simulink library "libAeroCoeffCalcs"  (R2020b)
settings: Solver=VariableStepAuto  StartTime=0.0  StopTime=10.0  RelTol=1e-3
undefined symbols (not defined in the file): data
libraries: aerolibconvert2 x2
settings Model: Creator=caatay  LastModifiedBy=caatay

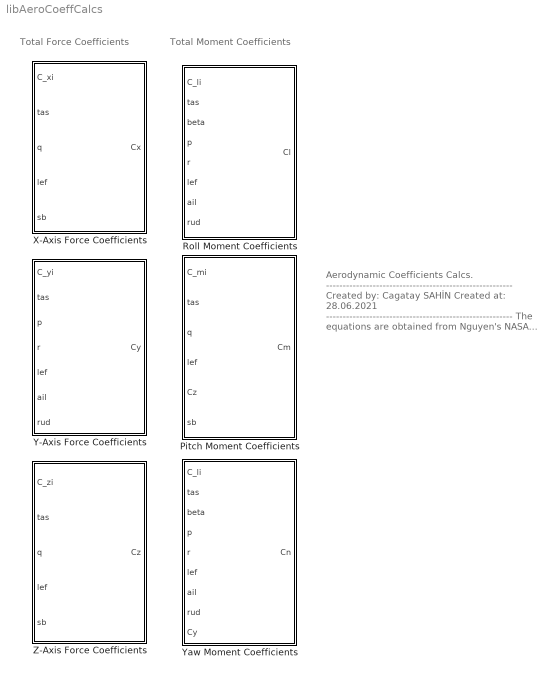
== system libAeroCoeffCalcs ==
  note: Aerodynamic Coefficients Calcs.
      | --------------------------------------------------------
      | Created by: Cagatay SAHİN
      | Created at: 28.06.2021
      | --------------------------------------------------------
      | The equations are obtained from
      | Nguyen's NASA works.
      | The reference article can be found in
      | "references folder".
      | --------------------------------------------------------
      | for question:
      | cagataysahin44@gmail.com
  note: Total Moment Coefficients
  note: Total Force Coefficients
  Pitch Moment Coefficients : Subsystem  mask(Aerodynamic Model - Total Coefficient Calculations - Total Pitch Moment Body Aerodynamic Coefficient){cbar=data.acSpec.wing.cbar, xcg=data.acSpec.fusalage.x_cg, xcg_ref=data.acSpec.fusalage.x_cg_ref}
      mask prompts: cbar "Mean Aerodynamic Chord"; xcg "X-axis center of gravity"; xcg_ref "Nominal X-axis center of gravity"
      mask help: Aircraft's total pitch moment aerodynamic coefficient calculations with using state variables and control inputs.
      mask Help:
      | This block is used for obtain total pitch moment coefficient with using state and control inputs.
      | -------------------------------------------------------------------------------------------------------------------------------------------------
      | Inputs of the function:
      | 	Coefficients C_{m}s: Pitch Moment whole aerodynamic coefficients at specific conditions.
      | 	tas: True air speed in [ft/s].
      | 	q: Body axis angular rate (pitch) in [rad/s].
      | 	lef: Leading edge flap deflection in [deg].
      | 	C_{z}: Z-Axis total aeodynamic coefficient.
      | Output of the function:
      | 	C_{m}: Pitch Moment total aerodynamic coefficient.
      | -------------------------------------------------------------------------------------------------------------------------------------------------
      | All equations can be found in Steven's text book. Reference can be found in "literature" subfolder.
      | for question: "cagataysahin44@gmail.com"
      mask Display:
      | port_label('input',1,'C_{m_{i}}','texmode','on');
      | port_label('input',2,'V_{tas}','texmode','on');
      | port_label('input',3,'q','texmode','on');
      | port_label('input',4,'\delta_{lef}','texmode','on');
      | port_label('input',5,'C_{z}','texmode','on');
      | port_label('input',6,'\delta_{sb}','texmode','on');
      | 
      | port_label('output',1,'C_{m}','texmode','on');
  Roll Moment Coefficients : Subsystem  mask(Aerodynamic Model - Total Coefficient Calculations - Total Roll Moment Body Aerodynamic Coefficient){b=data.acSpec.wing.b}
      mask prompts: b "Wing Span"
      mask help: Aircraft's total roll moment aerodynamic coefficient calculations with using state variables and control input
      mask Help:
      | This block is used for obtain total roll moment aerodynamic force coefficient. The equations are taken from Steven's textbook.,
      | -------------------------------------------------------------------------------------------------------------------------------------------------
      | Inputs of the function:
      | 	Coefficients C_{l}s: Roll moment whole aerodynamic coefficients at specific conditions.
      | 	tas: True air speed in [ft/s].
      |  	beta: Sideslip angle in [rad].
      | 	p: Body axis angular rate (roll) in [rad/s].
      | 	r: Body axis angular rate (yaw) in [rad/s].
      | 	lef: Leading edge flap deflection in [deg].
      | 	ail: Aileron deflection in [deg].
      | 	rud: Rudder deflection in [deg].
      | Output of the function:
      | 	C_{l}: Roll moment aerodynamic coefficient.
      | -------------------------------------------------------------------------------------------------------------------------------------------------
      | All equations can be found in Steven's text book. Reference can be found in "literature" subfolder.
      | for question: "cagataysahin44@gmail.com"
      mask Display:
      | port_label('input',1,'C_{l_{i}}','texmode','on');
      | port_label('input',2,'V_{tas}','texmode','on');
      | port_label('input',3,'\beta','texmode','on');
      | port_label('input',4,'p','texmode','on');
      | port_label('input',5,'r','texmode','on');
      | port_label('input',6,'\delta_{lef}','texmode','on');
      | port_label('input',7,'\delta_{ail}','texmode','on');
      | port_label('input',8,'\delta_{rud}','texmode','on');
      | 
      | port_label('output',1,'C_{l}','texmode','on');
  X-Axis Force Coefficients : Subsystem  mask(Aerodynamic Model - Total Coefficient Calculations - Total X-Axis Body Aerodynamic Coefficient){cbar=data.acSpec.wing.cbar}
      mask prompts: cbar "Mean Aerodynamic Chord"
      mask help: Aircraft's total X-Axis aerodynamic coefficient calculations with using state variables and control inputs.
      mask Help:
      | This block is used for obtain total x-axis aerodynamic force coefficient with using state and control inputs.
      | -------------------------------------------------------------------------------------------------------------------------------------------------
      | Inputs of the function:
      | 	Coefficients C_{x}s: X-Axis whole aerodynamic coefficients at specific conditions.
      | 	tas: True air speed in [ft/s].
      | 	q: Body axis angular rate (pitch) in [rad/s].
      | 	lef: Leading edge flap deflection in [deg].
      | Output of the function:
      | 	C_{x}: X-Axis total aerodynamic coefficient.
      | -------------------------------------------------------------------------------------------------------------------------------------------------
      | All equations can be found in Steven's text book. Reference can be found in "literature" subfolder.
      | for question: "cagataysahin44@gmail.com"
      mask Display:
      | port_label('input',1,'C_{x_{i}}','texmode','on');
      | port_label('input',2,'V_{tas}','texmode','on');
      | port_label('input',3,'q','texmode','on');
      | port_label('input',4,'\delta_{lef}','texmode','on');
      | port_label('input',5,'\delta_{sb}','texmode','on');
      | 
      | port_label('output',1,'C_{x}','texmode','on');
  Y-Axis Force Coefficients : Subsystem  mask(Aerodynamic Model - Total Coefficient Calculations - Total Y-Axis Body Aerodynamic Coefficient){b=data.acSpec.wing.b}
      mask prompts: b "Wing Span"
      mask help: Aircraft's total Y-Axis aerodynamic coefficient calculations with using state variables and control inputs.
      mask Help:
      | This block is used for obtain total x-axis aerodynamic force coefficient with using state and control inputs.
      | -------------------------------------------------------------------------------------------------------------------------------------------------
      | Inputs of the function:
      | 	Coefficients C_{y}s: Y-Axis whole aerodynamic coefficients at specific conditions.
      | 	tas: True air speed in [ft/s].
      | 	p: Body axis angular rate (y-axis) in [rad/s].
      | 	r: Body axis angular rate (y-axis) in [rad/s].
      | 	lef: Leading edge flap deflection in [deg].
      | 	ail: Aileron deflection in [deg].
      | 	rud: Rudder deflection in [deg].
      | Output of the function:
      | 	C_{y}: Y-axis total aerodynamic coefficient.
      | -------------------------------------------------------------------------------------------------------------------------------------------------
      | All equations can be found in Steven's text book. Reference can be found in "literature" subfolder.
      | for question: "cagataysahin44@gmail.com"
      mask Display:
      | port_label('input',1,'C_{y_{i}}','texmode','on');
      | port_label('input',2,'V_{tas}','texmode','on');
      | port_label('input',3,'p','texmode','on');
      | port_label('input',4,'r','texmode','on');
      | port_label('input',5,'\delta_{lef}','texmode','on');
      | port_label('input',6,'\delta_{ail}','texmode','on');
      | port_label('input',7,'\delta_{rud}','texmode','on');
      | 
      | port_label('output',1,'C_{y}','texmode','on');
  Yaw Moment Coefficients : Subsystem  mask(Aerodynamic Model - Total Coefficient Calculations - Total Yaw Moment Body Aerodynamic Coefficient){b=data.acSpec.wing.b, xcg=data.acSpec.fusalage.x_cg, xcg_ref=data.acSpec.fusalage.x_cg_ref, cbar=data.acSpec.wing.cbar}
      mask prompts: b "Wing Span"; xcg "Center of Gravity"; xcg_ref "Nominal Center of Gravity"; cbar "Mean Aerodynamic Chord"
      mask help: Aircraft's total yaw moment aerodynamic coefficient calculations with using state variables and control inputs.
      mask Help:
      | This block is used for obtain total yaw moment aerodynamic force coefficient. The equations are taken from Steven's textbook.,
      | -------------------------------------------------------------------------------------------------------------------------------------------------
      | Inputs of the function:
      | 	Coefficients C_{n}s: Yaw moment whole aerodynamic coefficients at specific conditions.
      | 	tas: True air speed in [ft/s].
      |  	beta: Sideslip angle in [rad].
      | 	p: Body axis angular rate (roll) in [rad/s].
      | 	r: Body axis angular rate (yaw) in [rad/s].
      | 	lef: Leading edge flap deflection in [deg].
      | 	ail: Aileron deflection in [deg].
      | 	rud: Rudder deflection in [deg].
      | 	C_{y}: Total Y-Axis aerodynamic coefficient.
      | Output of the function:
      | 	C_{n}: Yaw moment aerodynamic coefficient.
      | -------------------------------------------------------------------------------------------------------------------------------------------------
      | All equations can be found in Steven's text book. Reference can be found in "literature" subfolder.
      | for question: "cagataysahin44@gmail.com"
      mask Display:
      | port_label('input',1,'C_{n_{i}}','texmode','on');
      | port_label('input',2,'V_{tas}','texmode','on');
      | port_label('input',3,'\beta','texmode','on');
      | port_label('input',4,'p','texmode','on');
      | port_label('input',5,'r','texmode','on');
      | port_label('input',6,'\delta_{lef}','texmode','on');
      | port_label('input',7,'\delta_{ail}','texmode','on');
      | port_label('input',8,'\delta_{rud}','texmode','on');
      | port_label('input',9,'C_{y}','texmode','on');
      | 
      | port_label('output',1,'C_{n}','texmode','on');
  Z-Axis Force Coefficients : Subsystem  mask(Aerodynamic Model - Total Coefficient Calculations - Total Z-Axis Body Aerodynamic Coefficient){cbar=data.acSpec.wing.cbar}
      mask prompts: cbar "Mean Aerodynamic Chord"
      mask help: Aircraft's total Z-Axis aerodynamic coefficient calculations with using state variables and control inputs.
      mask Help:
      | This block is used for obtain total z-axis aerodynamic force coefficient with using state and control inputs.
      | -------------------------------------------------------------------------------------------------------------------------------------------------
      | Inputs of the function:
      | 	Coefficients C_{z}s: Z-Axis whole aerodynamic coefficients at specific conditions.
      | 	tas: True air speed in [ft/s].
      | 	q: Body axis angular rate (pitch) in [rad/s].
      | 	lef: Leading edge flap deflection in [deg].
      | Output of the function:
      | 	C_{z}: X-Axis total aerodynamic coefficient.
      | -------------------------------------------------------------------------------------------------------------------------------------------------
      | All equations can be found in Steven's text book. Reference can be found in "literature" subfolder.
      | for question: "cagataysahin44@gmail.com"
      mask Display:
      | port_label('input',1,'C_{z_{i}}','texmode','on');
      | port_label('input',2,'V_{tas}','texmode','on');
      | port_label('input',3,'q','texmode','on');
      | port_label('input',4,'\delta_{lef}','texmode','on');
      | port_label('input',5,'\delta_{sb}','texmode','on');
      | 
      | port_label('output',1,'C_{z}','texmode','on');

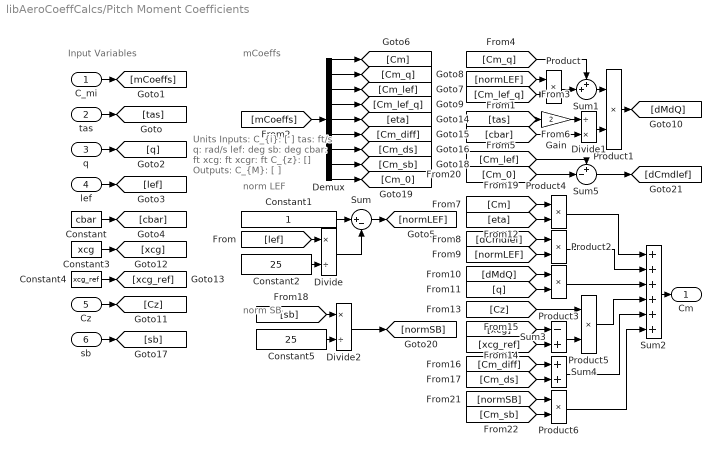
== system libAeroCoeffCalcs/Pitch Moment Coefficients ==
  note: Units
      | Inputs:
      | C_{i}: [ ]
      | tas: ft/s
      | q: rad/s
      | lef: deg
      | sb: deg
      | cbar: ft
      | xcg: ft
      | xcgr: ft
      | C_{z}: []
      | Outputs:
      | C_{M}: [ ]
  note: mCoeffs
  note: Input Variables
  note: norm LEF
  note: norm SB
  C_mi : Inport
  tas : Inport  Port=2
  q : Inport  Port=3
  lef : Inport  Port=4
  Cz : Inport  Port=5
  sb : Inport  Port=6
  Constant : Constant  Value=cbar
  Constant1 : Constant
  Constant2 : Constant  Value=25
  Constant3 : Constant  Value=xcg
  Constant4 : Constant  Value=xcg_ref
  Constant5 : Constant  Value=25
  Demux : Demux  Outputs=9
  Divide : Product  Inputs=*/
  Divide1 : Product  Inputs=/*
  Divide2 : Product  Inputs=*/
  Gain : Gain  Gain=2
  Product{,1..6} (7 alike) : Product
  Sum : Sum  Inputs=|+-
  Sum1 : Sum  Inputs=++|
  Sum2 : Sum  Inputs=++++++
  Sum3 : Sum  Inputs=-+
  Sum4 : Sum
  Sum5 : Sum  Inputs=+-|
  Cm : Outport  VectorParamsAs1DForOutWhenUnconnected=off
  wires:
  Product2/1 -> Sum2/2
  [Cm] -> Product4/1
  [normLEF] -> Product2/2
  [dCmdlef] -> Product2/1
  [Cm_q] -> Sum1/1
  Sum2/1 -> Cm/1
  Divide1/1 -> Product1/2
  Gain/1 -> Divide1/1
  Sum1/1 -> Product1/1
  [Cm_lef_q] -> Product/2
  [normLEF] -> Product/1
  [mCoeffs] -> Demux/1
  Product1/1 -> [dMdQ]
  Demux/3 -> [Cm_lef]
  [dMdQ] -> Product3/1
  Demux/1 -> [Cm]
  Demux/4 -> [Cm_lef_q]
  [lef] -> Divide/1
  Sum/1 -> [normLEF]
  Product3/1 -> Sum2/3
  [tas] -> Gain/1
  [cbar] -> Divide1/2
  Demux/2 -> [Cm_q]
  Product/1 -> Sum1/2
  lef/1 -> [lef]
  Constant/1 -> [cbar]
  Constant2/1 -> Divide/2
  Constant1/1 -> Sum/1
  [q] -> Product3/2
  C_mi/1 -> [mCoeffs]
  Divide/1 -> Sum/2
  q/1 -> [q]
  tas/1 -> [tas]
  Cz/1 -> [Cz]
  Constant3/1 -> [xcg]
  Constant4/1 -> [xcg_ref]
  Demux/7 -> [Cm_ds]
  Demux/6 -> [Cm_diff]
  Demux/5 -> [eta]
  [eta] -> Product4/2
  Product4/1 -> Sum2/1
  [xcg_ref] -> Sum3/2
  [xcg] -> Sum3/1
  [Cz] -> Product5/1
  Sum3/1 -> Product5/2
  [Cm_ds] -> Sum4/2
  [Cm_diff] -> Sum4/1
  Sum4/1 -> Sum2/5
  Product5/1 -> Sum2/4
  Demux/8 -> [Cm_sb]
  Demux/9 -> [Cm_0]
  Constant5/1 -> Divide2/2
  [sb] -> Divide2/1
  Divide2/1 -> [normSB]
  Sum5/1 -> [dCmdlef]
  [Cm_sb] -> Product6/2
  [normSB] -> Product6/1
  Product6/1 -> Sum2/6
  [Cm_0] -> Sum5/2
  [Cm_lef] -> Sum5/1
  sb/1 -> [sb]

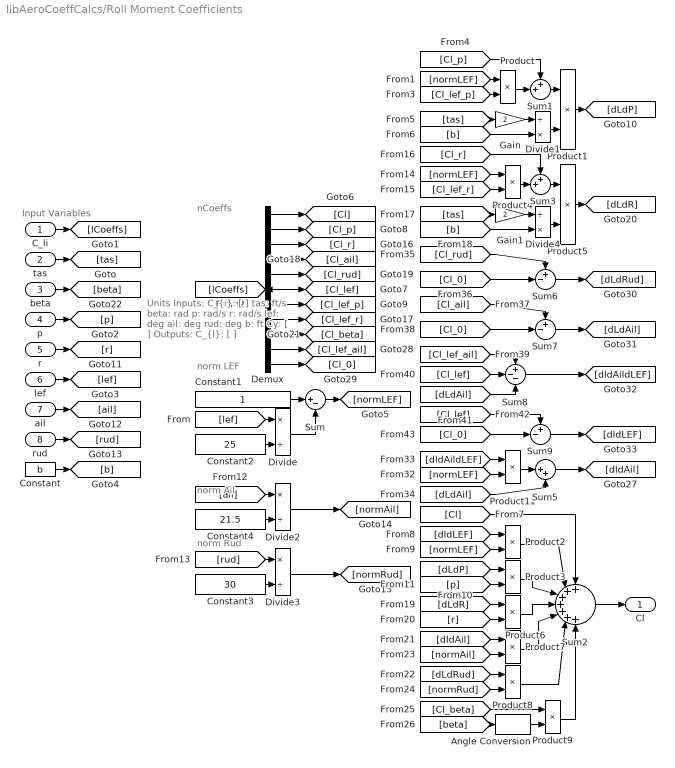
== system libAeroCoeffCalcs/Roll Moment Coefficients ==
  note: Units
      | Inputs:
      | C_{i}: [ ]
      | tas: ft/s
      | beta: rad
      | p: rad/s
      | r: rad/s
      | lef: deg
      | ail: deg
      | rud: deg
      | b: ft
      | Cy: [ ]
      | Outputs:
      | C_{l}: [ ]
  note: norm Ail
  note: norm LEF
  note: nCoeffs
  note: Input Variables
  note: norm Rud
  C_li : Inport
  tas : Inport  Port=2
  beta : Inport  Port=3
  p : Inport  Port=4
  r : Inport  Port=5
  lef : Inport  Port=6
  ail : Inport  Port=7
  rud : Inport  Port=8
  Angle Conversion : aerolibconvert2/Angle Conversion  IU=rad  OU=deg
  Constant : Constant  Value=b
  Constant1 : Constant
  Constant2 : Constant  Value=25
  Constant3 : Constant  Value=30
  Constant4 : Constant  Value=21.5
  Demux : Demux  Outputs=11
  Divide : Product  Inputs=*/
  Divide1 : Product  Inputs=/*
  Divide2 : Product  Inputs=*/
  Divide3 : Product  Inputs=*/
  Divide4 : Product  Inputs=/*
  Gain : Gain  Gain=2
  Gain1 : Gain  Gain=2
  Product{,1..9,11} (11 alike) : Product
  Sum : Sum  Inputs=|+-
  Sum1 : Sum  Inputs=++|
  Sum2 : Sum  Inputs=+++++++
  Sum3 : Sum  Inputs=++|
  Sum5 : Sum  Inputs=|++
  Sum6 : Sum  Inputs=+-|
  Sum7 : Sum  Inputs=+-|
  Sum8 : Sum  Inputs=+--
  Sum9 : Sum  Inputs=+-|
  Cl : Outport  VectorParamsAs1DForOutWhenUnconnected=off
  wires:
  [Cl_lef_ail] -> Sum8/1
  [Cl_lef] -> Sum9/1
  [dLdAil] -> Sum8/3
  Sum7/1 -> [dLdAil]
  [Cl_ail] -> Sum7/1
  [Cl_lef] -> Sum8/2
  [Cl_0] -> Sum9/2
  Sum9/1 -> [dldLEF]
  [Cl_0] -> Sum6/2
  [Cl_rud] -> Sum6/1
  Demux/11 -> [Cl_0]
  [lCoeffs] -> Demux/1
  Constant3/1 -> Divide3/2
  [normRud] -> Product8/2
  beta/1 -> [beta]
  r/1 -> [r]
  [dldLEF] -> Product2/1
  Demux/8 -> [Cl_lef_r]
  [Cl_0] -> Sum7/2
  Gain1/1 -> Divide4/1
  Demux/6 -> [Cl_lef]
  lef/1 -> [lef]
  Sum3/1 -> Product5/1
  ail/1 -> [ail]
  Divide3/1 -> [normRud]
  Product4/1 -> Sum3/2
  [Cl_r] -> Sum3/1
  [normAil] -> Product7/2
  [tas] -> Gain/1
  Product6/1 -> Sum2/4
  [dLdR] -> Product6/1
  Product2/1 -> Sum2/2
  [Cl_p] -> Sum1/1
  Demux/2 -> [Cl_p]
  Sum6/1 -> [dLdRud]
  Product7/1 -> Sum2/5
  Divide/1 -> Sum/2
  Demux/5 -> [Cl_rud]
  Constant2/1 -> Divide/2
  Gain/1 -> Divide1/1
  Product3/1 -> Sum2/3
  [rud] -> Divide3/1
  [normLEF] -> Product/1
  [r] -> Product6/2
  Divide1/1 -> Product1/2
  p/1 -> [p]
  [b] -> Divide4/2
  [lef] -> Divide/1
  Demux/9 -> [Cl_beta]
  Divide2/1 -> [normAil]
  Product/1 -> Sum1/2
  [Cl_lef_p] -> Product/2
  [b] -> Divide1/2
  C_li/1 -> [lCoeffs]
  Product9/1 -> Sum2/7
  Product5/1 -> [dLdR]
  Demux/10 -> [Cl_lef_ail]
  Sum8/1 -> [dldAildLEF]
  [dLdAil] -> Sum5/2
  Divide4/1 -> Product5/2
  [dldAildLEF] -> Product11/1
  [p] -> Product3/2
  [dLdP] -> Product3/1
  Demux/4 -> [Cl_ail]
  [tas] -> Gain1/1
  [Cl_lef_r] -> Product4/2
  rud/1 -> [rud]
  Product11/1 -> Sum5/1
  [dldAil] -> Product7/1
  Sum/1 -> [normLEF]
  [Cl] -> Sum2/1
  [normLEF] -> Product11/2
  Constant/1 -> [b]
  Sum1/1 -> Product1/1
  Constant1/1 -> Sum/1
  [normLEF] -> Product4/1
  Constant4/1 -> Divide2/2
  Product8/1 -> Sum2/6
  [ail] -> Divide2/1
  Demux/7 -> [Cl_lef_p]
  Demux/3 -> [Cl_r]
  [Cl_beta] -> Product9/1
  [dLdRud] -> Product8/1
  Sum2/1 -> Cl/1
  tas/1 -> [tas]
  Product1/1 -> [dLdP]
  [normLEF] -> Product2/2
  Sum5/1 -> [dldAil]
  Demux/1 -> [Cl]
  [beta] -> Angle Conversion/1
  Angle Conversion/1 -> Product9/2

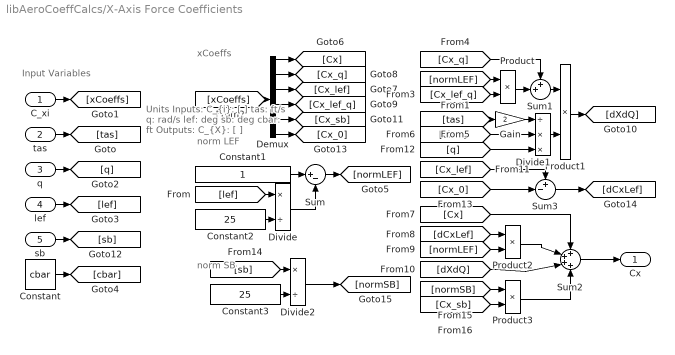
== system libAeroCoeffCalcs/X-Axis Force Coefficients ==
  note: norm LEF
  note: Units
      | Inputs:
      | C_{i}: [ ]
      | tas: ft/s
      | q: rad/s
      | lef: deg
      | sb: deg
      | cbar: ft
      | Outputs:
      | C_{X}: [ ]
  note: Input Variables
  note: xCoeffs
  note: norm SB
  C_xi : Inport
  tas : Inport  Port=2
  q : Inport  Port=3
  lef : Inport  Port=4
  sb : Inport  Port=5
  Constant : Constant  Value=cbar
  Constant1 : Constant
  Constant2 : Constant  Value=25
  Constant3 : Constant  Value=25
  Demux : Demux  Outputs=6
  Divide : Product  Inputs=*/
  Divide1 : Product  Inputs=/**
  Divide2 : Product  Inputs=*/
  Gain : Gain  Gain=2
  Product{,1..3} (4 alike) : Product
  Sum : Sum  Inputs=|+-
  Sum1 : Sum  Inputs=++|
  Sum2 : Sum  Inputs=++++
  Sum3 : Sum  Inputs=+-|
  Cx : Outport  VectorParamsAs1DForOutWhenUnconnected=off
  wires:
  tas/1 -> [tas]
  C_xi/1 -> [xCoeffs]
  q/1 -> [q]
  lef/1 -> [lef]
  Constant/1 -> [cbar]
  Constant2/1 -> Divide/2
  [lef] -> Divide/1
  Divide/1 -> Sum/2
  Constant1/1 -> Sum/1
  Sum/1 -> [normLEF]
  [xCoeffs] -> Demux/1
  Demux/1 -> [Cx]
  Demux/2 -> [Cx_q]
  Demux/3 -> [Cx_lef]
  Demux/4 -> [Cx_lef_q]
  [normLEF] -> Product/1
  [Cx_lef_q] -> Product/2
  [Cx_q] -> Sum1/1
  Product/1 -> Sum1/2
  [tas] -> Gain/1
  Gain/1 -> Divide1/1
  [cbar] -> Divide1/2
  Divide1/1 -> Product1/2
  Sum1/1 -> Product1/1
  Product1/1 -> [dXdQ]
  [normLEF] -> Product2/2
  [dCxLef] -> Product2/1
  Product2/1 -> Sum2/2
  [dXdQ] -> Sum2/3
  [Cx] -> Sum2/1
  Sum2/1 -> Cx/1
  Demux/5 -> [Cx_sb]
  sb/1 -> [sb]
  [q] -> Divide1/3
  Demux/6 -> [Cx_0]
  [Cx_lef] -> Sum3/1
  [Cx_0] -> Sum3/2
  Sum3/1 -> [dCxLef]
  [sb] -> Divide2/1
  Constant3/1 -> Divide2/2
  Divide2/1 -> [normSB]
  [Cx_sb] -> Product3/2
  [normSB] -> Product3/1
  Product3/1 -> Sum2/4

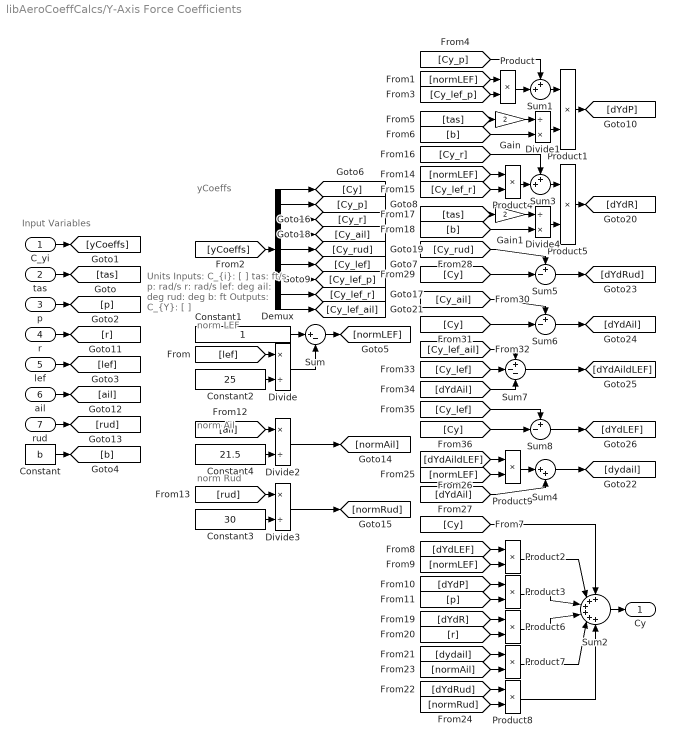
== system libAeroCoeffCalcs/Y-Axis Force Coefficients ==
  note: Units
      | Inputs:
      | C_{i}: [ ]
      | tas: ft/s
      | p: rad/s
      | r: rad/s
      | lef: deg
      | ail: deg
      | rud: deg
      | b: ft
      | Outputs:
      | C_{Y}: [ ]
  note: yCoeffs
  note: Input Variables
  note: norm LEF
  note: norm Ail
  note: norm Rud
  C_yi : Inport
  tas : Inport  Port=2
  p : Inport  Port=3
  r : Inport  Port=4
  lef : Inport  Port=5
  ail : Inport  Port=6
  rud : Inport  Port=7
  Constant : Constant  Value=b
  Constant1 : Constant
  Constant2 : Constant  Value=25
  Constant3 : Constant  Value=30
  Constant4 : Constant  Value=21.5
  Demux : Demux  Outputs=9
  Divide : Product  Inputs=*/
  Divide1 : Product  Inputs=/*
  Divide2 : Product  Inputs=*/
  Divide3 : Product  Inputs=*/
  Divide4 : Product  Inputs=/*
  Gain : Gain  Gain=2
  Gain1 : Gain  Gain=2
  Product{,1..9} (10 alike) : Product
  Sum : Sum  Inputs=|+-
  Sum1 : Sum  Inputs=++|
  Sum2 : Sum  Inputs=++++++
  Sum3 : Sum  Inputs=++|
  Sum4 : Sum  Inputs=|++
  Sum5 : Sum  Inputs=+-|
  Sum6 : Sum  Inputs=+-|
  Sum7 : Sum  Inputs=+--
  Sum8 : Sum  Inputs=+-|
  Cy : Outport  VectorParamsAs1DForOutWhenUnconnected=off
  wires:
  Demux/2 -> [Cy_p]
  Demux/1 -> [Cy]
  lef/1 -> [lef]
  [dYdLEF] -> Product2/1
  Sum1/1 -> Product1/1
  [Cy_lef_p] -> Product/2
  Constant2/1 -> Divide/2
  Gain/1 -> Divide1/1
  Divide1/1 -> Product1/2
  [normLEF] -> Product2/2
  C_yi/1 -> [yCoeffs]
  [b] -> Divide1/2
  [yCoeffs] -> Demux/1
  Product1/1 -> [dYdP]
  [normLEF] -> Product/1
  Constant/1 -> [b]
  Sum/1 -> [normLEF]
  tas/1 -> [tas]
  [lef] -> Divide/1
  Demux/7 -> [Cy_lef_p]
  p/1 -> [p]
  Divide/1 -> Sum/2
  Product/1 -> Sum1/2
  [Cy_p] -> Sum1/1
  [tas] -> Gain/1
  [dYdP] -> Product3/1
  Demux/6 -> [Cy_lef]
  [p] -> Product3/2
  Constant1/1 -> Sum/1
  r/1 -> [r]
  ail/1 -> [ail]
  rud/1 -> [rud]
  Divide2/1 -> [normAil]
  [ail] -> Divide2/1
  Constant4/1 -> Divide2/2
  Divide3/1 -> [normRud]
  Constant3/1 -> Divide3/2
  [rud] -> Divide3/1
  Demux/3 -> [Cy_r]
  Demux/8 -> [Cy_lef_r]
  Demux/5 -> [Cy_rud]
  Demux/4 -> [Cy_ail]
  [b] -> Divide4/2
  [normLEF] -> Product4/1
  Divide4/1 -> Product5/2
  [Cy_lef_r] -> Product4/2
  Sum3/1 -> Product5/1
  [tas] -> Gain1/1
  [Cy_r] -> Sum3/1
  Gain1/1 -> Divide4/1
  Product4/1 -> Sum3/2
  Product5/1 -> [dYdR]
  [r] -> Product6/2
  [dYdR] -> Product6/1
  [normRud] -> Product8/2
  [dYdRud] -> Product8/1
  [normAil] -> Product7/2
  [dydail] -> Product7/1
  Sum2/1 -> Cy/1
  Product6/1 -> Sum2/4
  Product3/1 -> Sum2/3
  Product2/1 -> Sum2/2
  [Cy] -> Sum2/1
  Product8/1 -> Sum2/6
  Product7/1 -> Sum2/5
  Demux/9 -> [Cy_lef_ail]
  [normLEF] -> Product9/2
  [dYdAildLEF] -> Product9/1
  Product9/1 -> Sum4/1
  [dYdAil] -> Sum4/2
  Sum4/1 -> [dydail]
  [Cy_rud] -> Sum5/1
  [Cy] -> Sum5/2
  Sum5/1 -> [dYdRud]
  [Cy] -> Sum6/2
  Sum6/1 -> [dYdAil]
  [Cy_ail] -> Sum6/1
  [Cy_lef_ail] -> Sum7/1
  [dYdAil] -> Sum7/3
  [Cy_lef] -> Sum7/2
  Sum7/1 -> [dYdAildLEF]
  Sum8/1 -> [dYdLEF]
  [Cy] -> Sum8/2
  [Cy_lef] -> Sum8/1

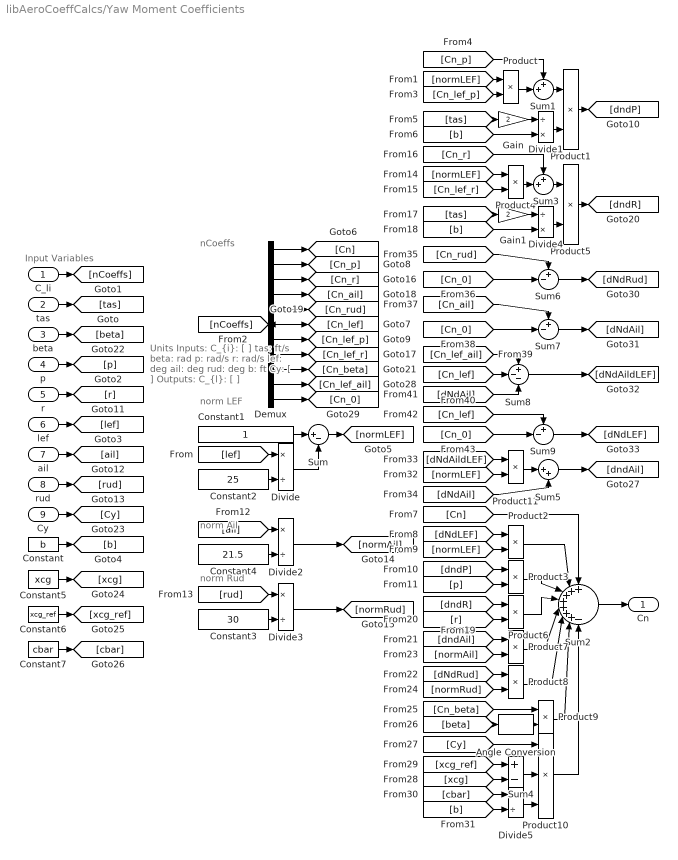
== system libAeroCoeffCalcs/Yaw Moment Coefficients ==
  note: Input Variables
  note: nCoeffs
  note: Units
      | Inputs:
      | C_{i}: [ ]
      | tas: ft/s
      | beta: rad
      | p: rad/s
      | r: rad/s
      | lef: deg
      | ail: deg
      | rud: deg
      | b: ft
      | Cy: [ ]
      | Outputs:
      | C_{l}: [ ]
  note: norm LEF
  note: norm Ail
  note: norm Rud
  C_li : Inport
  tas : Inport  Port=2
  beta : Inport  Port=3
  p : Inport  Port=4
  r : Inport  Port=5
  lef : Inport  Port=6
  ail : Inport  Port=7
  rud : Inport  Port=8
  Cy : Inport  Port=9
  Angle Conversion : aerolibconvert2/Angle Conversion  IU=rad  OU=deg
  Constant : Constant  Value=b
  Constant1 : Constant
  Constant2 : Constant  Value=25
  Constant3 : Constant  Value=30
  Constant4 : Constant  Value=21.5
  Constant5 : Constant  Value=xcg
  Constant6 : Constant  Value=xcg_ref
  Constant7 : Constant  Value=cbar
  Demux : Demux  Outputs=11
  Divide{,2..3,5} (4 alike) : Product  Inputs=*/
  Divide1 : Product  Inputs=/*
  Divide4 : Product  Inputs=/*
  Gain : Gain  Gain=2
  Gain1 : Gain  Gain=2
  Product{,1..9,11} (11 alike) : Product
  Product10 : Product  Inputs=3
  Sum : Sum  Inputs=|+-
  Sum1 : Sum  Inputs=++|
  Sum2 : Sum  Inputs=+++++++-
  Sum3 : Sum  Inputs=++|
  Sum4 : Sum  Inputs=+-
  Sum5 : Sum  Inputs=|++
  Sum6 : Sum  Inputs=+-|
  Sum7 : Sum  Inputs=+-|
  Sum8 : Sum  Inputs=+--
  Sum9 : Sum  Inputs=+-|
  Cn : Outport  VectorParamsAs1DForOutWhenUnconnected=off
  wires:
  Demux/9 -> [Cn_beta]
  Product9/1 -> Sum2/7
  C_li/1 -> [nCoeffs]
  [normLEF] -> Product2/2
  Product5/1 -> [dndR]
  [tas] -> Gain1/1
  [dndAil] -> Product7/1
  [dndP] -> Product3/1
  [normAil] -> Product7/2
  [b] -> Divide1/2
  [dNdLEF] -> Product2/1
  Product1/1 -> [dndP]
  [Cn_lef_p] -> Product/2
  Divide4/1 -> Product5/2
  Constant/1 -> [b]
  [Cn] -> Sum2/1
  Demux/3 -> [Cn_r]
  Divide1/1 -> Product1/2
  Product/1 -> Sum1/2
  Sum1/1 -> Product1/1
  [r] -> Product6/2
  Divide2/1 -> [normAil]
  tas/1 -> [tas]
  [lef] -> Divide/1
  p/1 -> [p]
  [normLEF] -> Product/1
  [b] -> Divide4/2
  [nCoeffs] -> Demux/1
  Demux/4 -> [Cn_ail]
  [rud] -> Divide3/1
  [dNdRud] -> Product8/1
  [normLEF] -> Product4/1
  Constant2/1 -> Divide/2
  Constant1/1 -> Sum/1
  Sum3/1 -> Product5/1
  [p] -> Product3/2
  Product3/1 -> Sum2/3
  [tas] -> Gain/1
  Product2/1 -> Sum2/2
  [Cn_p] -> Sum1/1
  [ail] -> Divide2/1
  Divide/1 -> Sum/2
  Gain/1 -> Divide1/1
  Demux/2 -> [Cn_p]
  [Cn_r] -> Sum3/1
  Constant4/1 -> Divide2/2
  Demux/7 -> [Cn_lef_p]
  Demux/8 -> [Cn_lef_r]
  Product4/1 -> Sum3/2
  Product8/1 -> Sum2/6
  [dndR] -> Product6/1
  Divide3/1 -> [normRud]
  Product7/1 -> Sum2/5
  Demux/5 -> [Cn_rud]
  Product6/1 -> Sum2/4
  Demux/1 -> [Cn]
  Constant3/1 -> Divide3/2
  Gain1/1 -> Divide4/1
  [Cn_lef_r] -> Product4/2
  [normRud] -> Product8/2
  beta/1 -> [beta]
  ail/1 -> [ail]
  rud/1 -> [rud]
  Demux/6 -> [Cn_lef]
  lef/1 -> [lef]
  Sum2/1 -> Cn/1
  Sum/1 -> [normLEF]
  r/1 -> [r]
  [Cn_beta] -> Product9/1
  Cy/1 -> [Cy]
  Constant6/1 -> [xcg_ref]
  Constant5/1 -> [xcg]
  Constant7/1 -> [cbar]
  [xcg_ref] -> Sum4/1
  [xcg] -> Sum4/2
  [cbar] -> Divide5/1
  [b] -> Divide5/2
  Sum4/1 -> Product10/2
  Divide5/1 -> Product10/3
  [Cy] -> Product10/1
  Product10/1 -> Sum2/8
  [dNdAil] -> Sum5/2
  Sum5/1 -> [dndAil]
  [normLEF] -> Product11/2
  Product11/1 -> Sum5/1
  [dNdAildLEF] -> Product11/1
  Demux/10 -> [Cn_lef_ail]
  Demux/11 -> [Cn_0]
  Sum8/1 -> [dNdAildLEF]
  [Cn_rud] -> Sum6/1
  Sum9/1 -> [dNdLEF]
  [Cn_0] -> Sum6/2
  [Cn_0] -> Sum7/2
  [Cn_lef] -> Sum8/2
  [Cn_0] -> Sum9/2
  Sum6/1 -> [dNdRud]
  Sum7/1 -> [dNdAil]
  [Cn_ail] -> Sum7/1
  [dNdAil] -> Sum8/3
  [Cn_lef_ail] -> Sum8/1
  [Cn_lef] -> Sum9/1
  [beta] -> Angle Conversion/1
  Angle Conversion/1 -> Product9/2

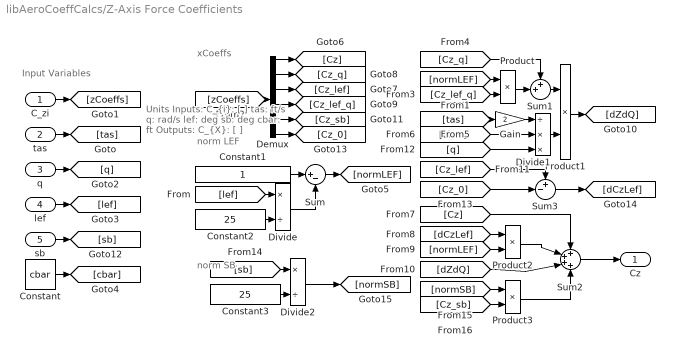
== system libAeroCoeffCalcs/Z-Axis Force Coefficients ==
  note: norm SB
  note: Input Variables
  note: norm LEF
  note: Units
      | Inputs:
      | C_{i}: [ ]
      | tas: ft/s
      | q: rad/s
      | lef: deg
      | sb: deg
      | cbar: ft
      | Outputs:
      | C_{X}: [ ]
  note: xCoeffs
  C_zi : Inport
  tas : Inport  Port=2
  q : Inport  Port=3
  lef : Inport  Port=4
  sb : Inport  Port=5
  Constant : Constant  Value=cbar
  Constant1 : Constant
  Constant2 : Constant  Value=25
  Constant3 : Constant  Value=25
  Demux : Demux  Outputs=6
  Divide : Product  Inputs=*/
  Divide1 : Product  Inputs=/**
  Divide2 : Product  Inputs=*/
  Gain : Gain  Gain=2
  Product{,1..3} (4 alike) : Product
  Sum : Sum  Inputs=|+-
  Sum1 : Sum  Inputs=++|
  Sum2 : Sum  Inputs=++++
  Sum3 : Sum  Inputs=+-|
  Cz : Outport  VectorParamsAs1DForOutWhenUnconnected=off
  wires:
  Product3/1 -> Sum2/4
  Demux/5 -> [Cz_sb]
  [Cz_0] -> Sum3/2
  [dZdQ] -> Sum2/3
  [Cz_sb] -> Product3/2
  Constant3/1 -> Divide2/2
  [normSB] -> Product3/1
  [Cz_q] -> Sum1/1
  [Cz_lef_q] -> Product/2
  [normLEF] -> Product/1
  [sb] -> Divide2/1
  Demux/4 -> [Cz_lef_q]
  [dCzLef] -> Product2/1
  Demux/1 -> [Cz]
  Divide1/1 -> Product1/2
  q/1 -> [q]
  Constant/1 -> [cbar]
  Constant1/1 -> Sum/1
  Sum3/1 -> [dCzLef]
  sb/1 -> [sb]
  [lef] -> Divide/1
  C_zi/1 -> [zCoeffs]
  Constant2/1 -> Divide/2
  Demux/2 -> [Cz_q]
  Product/1 -> Sum1/2
  [q] -> Divide1/3
  [Cz_lef] -> Sum3/1
  [zCoeffs] -> Demux/1
  [cbar] -> Divide1/2
  Gain/1 -> Divide1/1
  Demux/6 -> [Cz_0]
  [tas] -> Gain/1
  Sum2/1 -> Cz/1
  Sum/1 -> [normLEF]
  Product2/1 -> Sum2/2
  lef/1 -> [lef]
  Sum1/1 -> Product1/1
  Product1/1 -> [dZdQ]
  [normLEF] -> Product2/2
  [Cz] -> Sum2/1
  Divide2/1 -> [normSB]
  Demux/3 -> [Cz_lef]
  Divide/1 -> Sum/2
  tas/1 -> [tas]
